simulink model "GFLIB_Sqrt_BAM_F16"  (Simulink 7.3)
settings: Solver=ode45  StartTime=0.0  StopTime=10.0  RelTol=1e-3
settings Model: Creator=B17364  LastModifiedBy=B17364

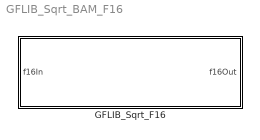
== system GFLIB_Sqrt_BAM_F16 ==
  GFLIB_Sqrt_F16 : Subsystem  mask(GFLIB_Sqrt_F16){}
      mask help: Bit accurate model of GFLIB_Sqrt function, which computes the square root of input value.
      mask init:
      | pos = get_param(gcb, 'Position');width = pos(3) - pos(1); height = pos(4) - pos(2);tX=width/2;tY=height*0.9;
      mask Display: color('black');port_label('input',1,'f16In');port_label('output',1,'f16Out');color('black');disp('GFLIB_Sqrt_F16');color('blue');text(tX,tY, 'BAM', 'horizontalAlignment', 'center');

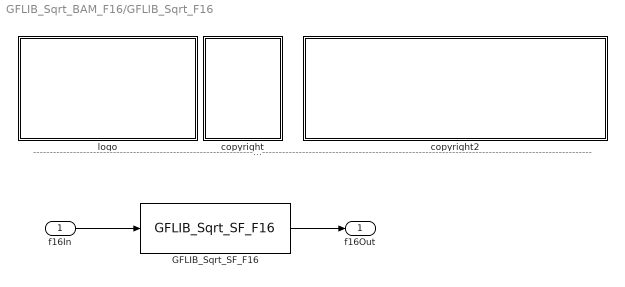
== system GFLIB_Sqrt_BAM_F16/GFLIB_Sqrt_F16 ==
  note: ---------------------------------------------------------------------------------------------------------------------------------------------------------------------------------------------------
  f16In : Inport  OutDataType=fixdt(1, 16)  OutScaling=2^0
  GFLIB_Sqrt_SF_F16 : S-Function  FunctionName=GFLIB_Sqrt_SF_F16  EnableBusSupport=off
  copyright : Subsystem
      mask Display: text(10,90,'FILE:');text(10,75,'DESRIPTION:')text(10,60,'COPYRIGHT:')text(10,45,'VERSION:')text(10,30,'DATE:')
  copyright2 : Subsystem
      mask Display: text(10,90,'GFLIB_Sqrt_BAM_F16.mdl');text(10,75,'Square root approximation.');text(10,60,'Freescale')text(10,45,'0.1');text(10,30,'12-Sep-2011');
  logo : Subsystem
      mask Display: image(imread('logo.jpg'))
  f16Out : Outport  OutDataType=fixdt(1, 16)  OutScaling=2^0
  wires:
  f16In/1 -> GFLIB_Sqrt_SF_F16/1
  GFLIB_Sqrt_SF_F16/1 -> f16Out/1

== system GFLIB_Sqrt_BAM_F16/GFLIB_Sqrt_F16/copyright ==

== system GFLIB_Sqrt_BAM_F16/GFLIB_Sqrt_F16/copyright2 ==

== system GFLIB_Sqrt_BAM_F16/GFLIB_Sqrt_F16/logo ==
